simulink model "vonkarman_generator"  (R2023a)
settings: Solver=ode4  StartTime=0.0  StopTime=12  FixedStep=0.00342875  RelTol=1e-3
undefined symbols (not defined in the file or in its folder): F, Light, MIL
libraries: aerolibwind2 x1
settings Model: Creator=elija  LastModifiedBy=elija

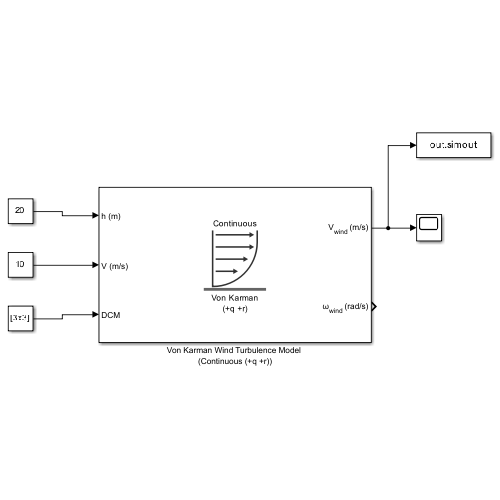
[thumbnail: Simulink's stored preview of the top-level diagram]
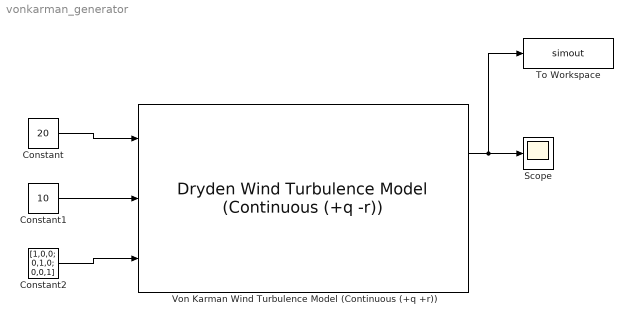
== system vonkarman_generator ==
  Constant : Constant  Value=20
  Constant1 : Constant  Value=10
  Constant2 : Constant  Value=[1,0,0; 0,1,0; 0,0,1]
  Scope : Scope
  To Workspace : ToWorkspace  VariableName=simout  SaveFormat=Timeseries  SampleTime=-1
  Von Karman Wind Turbulence Model (Continuous (+q +r)) : aerolibwind2/Dryden Wind Turbulence Model  (Continuous (+q -r))  units=Metric (MKS)  spec=MIL-F-8785C  model=Continuous Von Karman (+q +r)  W20=15  Wdeg=0  TurbProb=10^-2 - Light  L_high=762  Wingspan=1  ts=0.00342875  Seed=[13341 13342 13343 13344]  T_on=on
      settings: LibrarySourceBlock=|
      | aerolibwind2/Von Karman Wind Turbulence Model
      | (Continuous (+q +r))
  wires:
  Constant/1 -> Von Karman Wind Turbulence Model (Continuous (+q +r))/1
  Constant1/1 -> Von Karman Wind Turbulence Model (Continuous (+q +r))/2
  Constant2/1 -> Von Karman Wind Turbulence Model (Continuous (+q +r))/3
  Von Karman Wind Turbulence Model (Continuous (+q +r))/1 -> To Workspace/1, Scope/1
